simulink model "lowpass_equi_PAM"  (R2018a)
settings: Solver=ode45  StartTime=0.0  StopTime=1000  RelTol=1e-3  EnableMultiTasking=on
InitFcn:
  | lowpass_equi_PAM_ini;
undefined symbols (not defined in the file or in its folder): gcbh, j, rcfiltgaincompat
libraries: commnoisgen2 x2, commrandsrc2 x1, commdigbbndam3 x1, commsink2 x1, commutil2 x1, dspobslib x1, commfilt2 x1
settings Model: Creator=erban  LastModifiedBy=alumno
settings DataIOCC: LimitDataPoints=on  SaveFormat=Array  SignalLoggingSaveFormat=ModelDataLogs  SignalLoggingName=sigsOut
settings OptimizationCC: BooleanDataType=off
settings DebuggingCC: SaveWithParameterizedLinksMsg=none  UnderspecifiedInitializationDetection=Classic  MergeDetectMultiDrivingBlocksExec=none  SignalResolutionControl=TryResolveAllWithWarning  MultiTaskDSMMsg=warning  MultiTaskCondExecSysMsg=none
settings HardwareCC: ProdBitPerPointer=32  ProdBitPerSizeT=32  ProdBitPerPtrDiffT=32  ProdLargestAtomicFloat=None  ProdIntDivRoundTo=Undefined  ProdEndianess=Unspecified  ProdWordSize=32  ProdHWDeviceType=32-bit Generic  TargetUnknown=on
settings ModelReferenceCC: PropagateSignalLabelsOutOfModel=off
settings CodeAppCC: StateflowObjectComments=on
settings GRTTargetCC: TargetLangStandard=C89/C90 (ANSI)  CombineOutputUpdateFcns=off  GRTInterface=on
settings ConfigComp: CovMetricSettings=dw  CovHtmlReporting=on  CovSaveCumulativeToWorkspaceVar=on  CovSaveSingleToWorkspaceVar=on  CovExternalEMLEnable=off

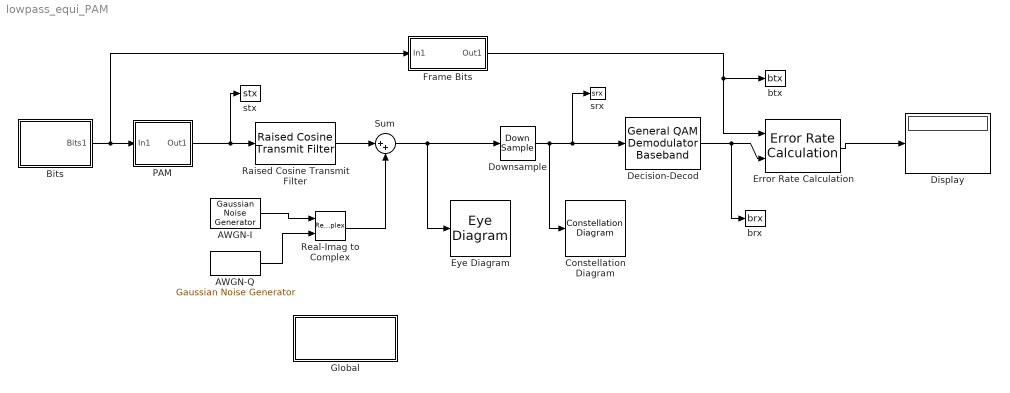
== system lowpass_equi_PAM ==
  AWGN-I : commnoisgen2/Gaussian Noise Generator  m=0  d=0.2  s=floor(60 * rand)+1  Ts=-1  frameBased=on  sampPerFrame=16  orient=off  outDataType=double
  AWGN-Q : commnoisgen2/Gaussian Noise Generator  m=0  d=0.2  s=floor(60 * rand)+1  Ts=-1  frameBased=on  sampPerFrame=16  orient=off  outDataType=double
  Bits : Subsystem
      mask Display: disp('11001010');
  Constellation Diagram : ConstellationDiagram
  Decision-Decod : commdigbbndam3/General QAM Demodulator Baseband  SigCon=[1+j,-1+j,1-j,-1-j]  OutType=Bit  DecType=Hard decision  VarSource=Dialog  Variance=1  outDtypeBit=Inherit via internal rule  outDtype=Inherit via internal rule  roundingMode=Floor  overflowMode=Wrap  OvFlMode=off  OvFlModeLastStrValue=off  sigConstWordLen=16  sigConstDataTypeStr=Inherit: Same word length as input  sigConstLastDataTypeStr=Inherit: Same word length as input  accum1WordLen=32  accum1FracLen=30  prodInWordLen=32  prodInFracLen=30  prodInDataTypeStr=Inherit: Same as accumulator 1  prodInLastDataTypeStr=Inherit: Same as accumulator 1  prodOutWordLen=32  prodOutFracLen=30  accum2WordLen=32  accum2FracLen=30  accum3WordLen=32  accum3FracLen=30  nsiWordLen=32  nsiFracLen=30  nsiDataTypeStr=Inherit: Same as accumulator 3  nsiLastDataTypeStr=Inherit: Same as accumulator 3  invn0WordLen=16  invn0FracLen=8  invn0DataTypeStr=Inherit: Same word length as input  invn0LastDataTypeStr=Inherit: Same word length as input  outputWordLen=32  outputFracLen=30
      settings: SourceProductName=Communications System Toolbox  SourceProductBaseCode=CM
  Display : Display
  Downsample : DownSample  N=16  RateOptions=Allow multirate processing
  Error Rate Calculation : commsink2/Error Rate Calculation  N=12  st_delay=32  cp_mode=Entire frame  subframe=[]  PMode=Port  WsName=ErrorVec  RsMode2=off  stop=off  numErr=100  maxBits=1e6
  Eye Diagram : EyeDiagram
  Frame Bits : Subsystem
      mask Display: disp('Buffer & \n Frame')
  Global : Subsystem  mask{NoiseVar=0.2, constellation=[1+j,-1+j,1-j,-1-j], Rb=1000}
      mask Display: disp('NoiseVar \n Constellation \n Rb')
  PAM : Subsystem  mask{cnstl=[1+j,-1+j,1-j,-1-j]}
      mask prompts: cnstl "Constelation"
      mask help: Codificador.
      mask Display: disp('Symbol \n Encoder');
  Raised Cosine Transmit Filter : commfilt2/Raised Cosine Transmit Filter  filtType=Normal  R=1  filtSpan=10  N=16  filterGain=rcfiltgaincompat(gcbh)  InputProcessing=Columns as channels (frame based)  RateOptions=Enforce single-rate processing  framing=Mute  checkCoeff=off  variableName=bbb  checkGain=Normalized  sampMode=Mute  saveAsFlag=0  currentFiltSpan=10  D=(10)/2  launchFVT=on  roundingMode=Floor  overflowMode=off  coeffDataTypeStr=Inherit: Same word length as input  coeffMin=[]  coeffMax=[]  coeffLastDataTypeStr=Inherit: Same word length as input  outputDataTypeStr=Inherit: Same as accumulator  outputMin=[]  outputMax=[]  outputLastDataTypeStr=Inherit: Same as accumulator
  Real-Imag to Complex : RealImagToComplex
  Sum : Sum  Inputs=|++  SaturateOnIntegerOverflow=on
  brx : ToWorkspace  VariableName=brx  SampleTime=-1
      settings: Save2DSignal=2-D array (concatenate along first dimension)
  btx : ToWorkspace  VariableName=btx  SampleTime=-1
      settings: Save2DSignal=2-D array (concatenate along first dimension)
  srx : ToWorkspace  VariableName=srx  SampleTime=-1
      settings: Save2DSignal=2-D array (concatenate along first dimension)
  stx : ToWorkspace  VariableName=stx  SampleTime=-1
      settings: Save2DSignal=2-D array (concatenate along first dimension)
  wires:
  PAM/1(Out1) -> stx/1, Raised Cosine Transmit Filter/1
  Raised Cosine Transmit Filter/1 -> Sum/1
  AWGN-I/1 -> Real-Imag to Complex/1
  AWGN-Q/1 -> Real-Imag to Complex/2
  Real-Imag to Complex/1 -> Sum/2
  Sum/1 -> Downsample/1, Eye Diagram/1
  Downsample/1 -> Constellation Diagram/1, srx/1, Decision-Decod/1
  Decision-Decod/1 -> brx/1, Error Rate Calculation/2
  Error Rate Calculation/1 -> Display/1
  Bits/1(Bits1) -> PAM/1(In1), Frame Bits/1(In1)
  Frame Bits/1(Out1) -> Error Rate Calculation/1, btx/1

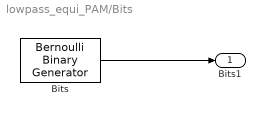
== system lowpass_equi_PAM/Bits ==
  Bits : commrandsrc2/Bernoulli Binary Generator  P=0.5  seed=floor(60 * rand)+1  Ts=0.001  frameBased=off  sampPerFrame=1  orient=off  outDataType=double
  Bits1 : Outport
  wires:
  Bits/1 -> Bits1/1

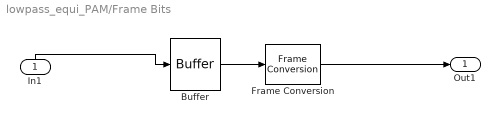
== system lowpass_equi_PAM/Frame Bits ==
  In1 : Inport
  Buffer : Buffer  N=32  OutputFrames=off
  Frame Conversion : FrameConversion
  Out1 : Outport
  wires:
  In1/1 -> Buffer/1
  Buffer/1 -> Frame Conversion/1
  Frame Conversion/1 -> Out1/1

== system lowpass_equi_PAM/Global ==

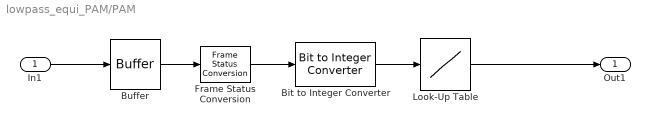
== system lowpass_equi_PAM/PAM ==
  In1 : Inport
  Bit to Integer Converter : commutil2/Bit to Integer Converter  nbits=log2(length(cnstl))  bitOrder=MSB first  signedOutputValues=Unsigned  outDtype=Inherit via internal rule  outDtypeSigned=Inherit via internal rule
  Buffer : Buffer  N=log2(length(cnstl))
  Frame Status Conversion : dspobslib/Frame Status Conversion  growRefPort=off  outframe=Sample-based
      settings: SourceProductName=DSP System Toolbox  SourceProductBaseCode=DS
  Look-Up Table : Lookup  InputValues=[0:length(cnstl)-1]  Table=cnstl  SaturateOnIntegerOverflow=on
  Out1 : Outport
  wires:
  Frame Status Conversion/1 -> Bit to Integer Converter/1
  In1/1 -> Buffer/1
  Buffer/1 -> Frame Status Conversion/1
  Look-Up Table/1 -> Out1/1
  Bit to Integer Converter/1 -> Look-Up Table/1
